simulink model "Exp_8"  (R2021a)
settings: Solver=VariableStepAuto  StartTime=0.0  StopTime=0.04  RelTol=1e-3
libraries: spsVoltageMeasurementLib x4, spsDiodeLib x2, spsLinearTransformerLib x1, spsACVoltageSourceLib x1, spsGroundLib x1, spsSeriesRLCBranchLib x1, spspowerguiLib x1
settings Model: Creator=Mehedi  LastModifiedBy=DCL
settings SolverCC: AlgebraicLoopSolver=TrustRegion
settings DataIOCC: ReturnWorkspaceOutputs=off
settings DebuggingCC: SFMachineParentedDataDiag=warning  ArithmeticOperatorsInVariantConditions=warning
settings SFSimCC: SimUseLocalCustomCode=off  CustomCodeUndefinedFunction=UseInterfaceOnly
settings RTWCC: RTWUseLocalCustomCode=off

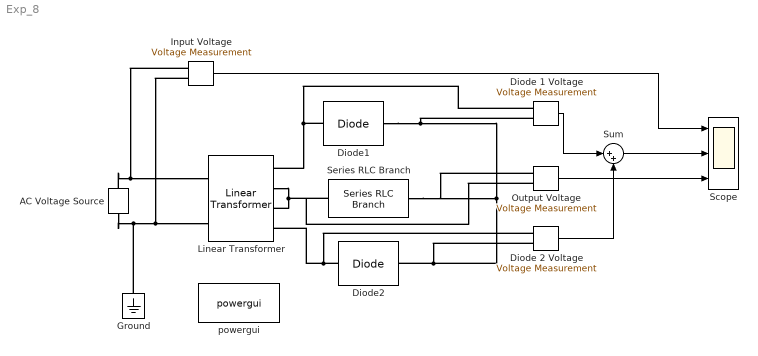
== system Exp_8 ==
  " Diode1" : spsDiodeLib/Diode  Ron=0  Lon=0  Vf=0  IC=0  UseSnubber=0  Rs=500  Cs=250e-9  Measurements=off
  " Diode2" : spsDiodeLib/Diode  Ron=0  Lon=0  Vf=0  IC=0  UseSnubber=0  Rs=500  Cs=250e-9  Measurements=off
  " Linear Transformer" : spsLinearTransformerLib/Linear Transformer  UNITS=pu  NominalPower=[ 250e6 50 ]  winding1="[ 30  0  0 ]"  winding2="[ 15  0  0 ]"  ThreeWindings=on  winding3="[ 15  0  0 ]"  RmLm=[inf inf]  Measurements=None  DataType=off
  " Scope" : Scope  NumInputPorts=3
  "  Diode 1 Voltage" : spsVoltageMeasurementLib/Voltage Measurement  PhasorSimulation=off  OutputType=Complex  PSBequivalent=0
  AC Voltage Source : spsACVoltageSourceLib/AC Voltage Source  Amplitude=240  Phase=0  Frequency=50  SampleTime=0  Measurements=None  BusType=swing  Pref=10e3  Qref=0  Qmin=-inf  Qmax=+inf
  Diode 2 Voltage : spsVoltageMeasurementLib/Voltage Measurement  PhasorSimulation=off  OutputType=Complex  PSBequivalent=0
  Ground : spsGroundLib/Ground  LConnTagsString=a
  Input Voltage : spsVoltageMeasurementLib/Voltage Measurement  PhasorSimulation=off  OutputType=Complex  PSBequivalent=0
  Output Voltage : spsVoltageMeasurementLib/Voltage Measurement  PhasorSimulation=off  OutputType=Complex  PSBequivalent=0
  Series RLC Branch : spsSeriesRLCBranchLib/Series RLC Branch  LConnTagsString=__new0  RConnTagsString=__new0  BranchType=R  Resistance=15  Inductance=1e-3  SetiL0=off  InitialCurrent=0  Capacitance=1e-6  Setx0=off  InitialVoltage=0  Measurements=None
  Sum : Sum  Inputs=|++
  powergui : spspowerguiLib/powergui  Priority=1  SimulationMode=Continuous  SampleTime=50e-6  frequency=60  Iterations=50  frequencyindice=50  Pbase=100e6  ErrMax=1e-4  UnitsV=kV  UnitsW=MW  buscounter=0  FunctionMessages=off  echomessages=off  EnableUseOfTLC=off  CurrentSourceSwitches=off  DisableSnubberDevices=off  DisableRonSwitches=off  DisableVfSwitches=off  DisplayEquations=off  AutomaticDiscreteSolvers=off  SolverType=Tustin/Backward Euler (TBE)  Interpol=off  ExternalGateDelay=off  methode=off  Ts=100  x0status=blocks  SPID=on  SwTol=0  HookPort=off  NonlinearTolerance=1e-4  nMaxIteration=100  ContinueOnMaxIteration=off  RestoreLinks=warning  ResistiveCurrentMeasurement=off  Frange=[0:2:500]  Ylog=off  Xlog=on  ShowGrid=off  save=off  variable=ZData  structure=0  ZoomFFT=off  StartTime=0.0  cycles=1  DisplayStyle=1  fundamental=60  FreqAxis=off  MaxFrequency=1000  frequencyindicesteady=1  RmsSteady=1  display=off
  wires:
  "  Diode 1 Voltage"/1 -> Sum/1
  Input Voltage/1 -> " Scope"/1
  Sum/1 -> " Scope"/2
  Output Voltage/1 -> " Scope"/3
  Diode 2 Voltage/1 -> Sum/2
  connections:
  " Linear Transformer"/RConn2 -- Output Voltage/LConn2 -- Series RLC Branch/LConn1 -- " Linear Transformer"/RConn3
  " Diode2"/LConn1 -- Diode 2 Voltage/LConn1 -- " Linear Transformer"/RConn4
  " Diode1"/RConn1 -- "  Diode 1 Voltage"/LConn2 -- Output Voltage/LConn1 -- Series RLC Branch/RConn1 -- Diode 2 Voltage/LConn2 -- " Diode2"/RConn1
  " Diode1"/LConn1 -- "  Diode 1 Voltage"/LConn1 -- " Linear Transformer"/RConn1
  AC Voltage Source/RConn1 -- Input Voltage/LConn1 -- " Linear Transformer"/LConn1
  AC Voltage Source/LConn1 -- Ground/LConn1 -- Input Voltage/LConn2 -- " Linear Transformer"/LConn2
